simulink model "linear_model"  (R2018b)
settings: Solver=VariableStepAuto  StartTime=0.0  StopTime=5  RelTol=1e-3
values from neighbouring files (symbols this model uses):
  A = [A11 A12 ... (first row only)    [makeBikeModel.m]
  B = [B11 B12 ... (first row only)    [makeBikeModel.m]
  C = eye(2)    [makeBikeModel.m]
  D = 0    [makeBikeModel.m]
  Lf = 2.56    [makeBikeModel.m]    (also in makePlants.m; tunePIDs.m = 0.55)
  Lr = 1.02    [makeBikeModel.m]    (also in makePlants.m; tunePIDs.m = 0.525)
libraries: simulink x1
settings Model: Creator=lachc  LastModifiedBy=lachc

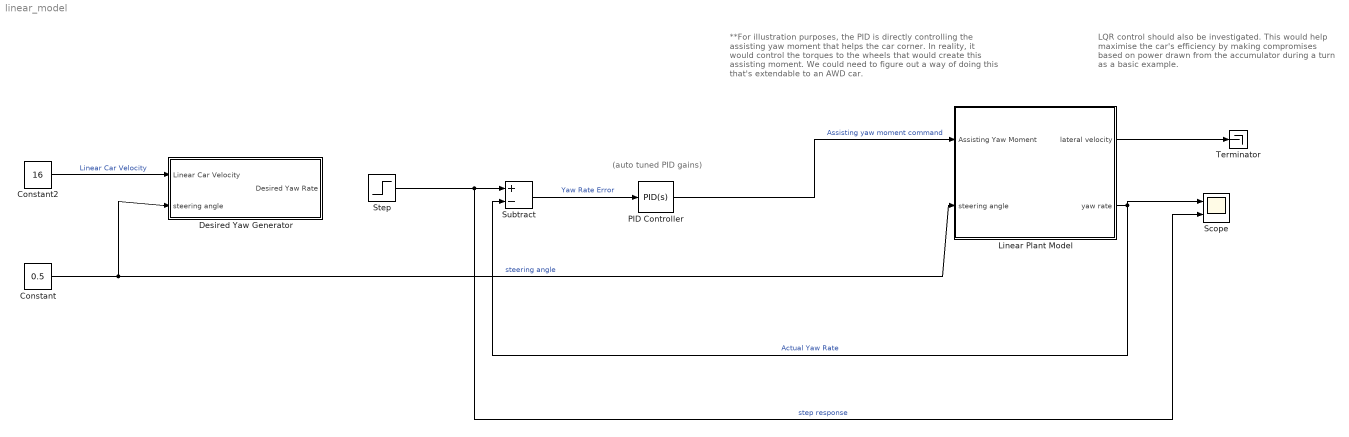
== system linear_model ==
  note: LQR control should also be investigated. This would help maximise the car's efficiency by making compromises based on power drawn from the accumulator during a turn as a basic example.
  note: **For illustration purposes, the PID is directly controlling the assisting yaw moment that helps the car corner. In reality, it would control the torques to the wheels that would create this assisting moment. We could need to figure out a way of doing this that's extendable to an AWD car.
  note: (auto tuned PID gains)
  Constant : Constant  Value=0.5
  Constant2 : Constant  Value=16
  Desired Yaw Generator : Subsystem
  Linear Plant Model : Subsystem
  PID Controller : simulink/Continuous/PID Controller  Controller=PID  Form=Parallel  TimeDomain=Continuous-time  SampleTime=-1  IntegratorMethod=Forward Euler  FilterMethod=Forward Euler  ControllerParametersSource=internal  P=140  I=2312  D=0.85  UseFilter=on  N=47  TunerSelectOption=Transfer Function Based (PID Tuner App)  InitialConditionSource=internal  InitialConditionForIntegrator=0  InitialConditionForFilter=0  DifferentiatorICPrevScaledInput=0  ExternalReset=none  TrackingMode=off  Kt=1  LimitOutput=off  UpperSaturationLimit=inf  LowerSaturationLimit=-inf  LinearizeAsGain=on  AntiWindupMode=none  Kb=1  POutMin=[]  POutMax=[]  IOutMin=[]  IOutMax=[]  DOutMin=[]  DOutMax=[]  NOutMin=[]  NOutMax=[]  SumOutMin=[]  SumOutMax=[]  SaturationOutMin=[]  SaturationOutMax=[]  PParamMin=[]  PParamMax=[]  IParamMin=[]  IParamMax=[]  DParamMin=[]  DParamMax=[]  NParamMin=[]  NParamMax=[]  KbParamMin=[]  KbParamMax=[]  KtParamMin=[]  KtParamMax=[]  KbOutMin=[]  KbOutMax=[]  KtOutMin=[]  KtOutMax=[]  IntegratorOutMin=[]  IntegratorOutMax=[]  FilterOutMin=[]  FilterOutMax=[]  SumI1OutMin=[]  SumI1OutMax=[]  SumI2OutMin=[]  SumI2OutMax=[]  SumI3OutMin=[]  SumI3OutMax=[]  SumI4OutMin=[]  SumI4OutMax=[]  SumDOutMin=[]  SumDOutMax=[]  DifferentiatorOutMin=[]  DifferentiatorOutMax=[]  FilterDiffOutCoefMin=[]  FilterDiffOutCoefMax=[]  ReciprocalOutMin=[]  ReciprocalOutMax=[]  SumDenOutMin=[]  SumDenOutMax=[]  SumNumOutMin=[]  SumNumOutMax=[]  DivideOutMin=[]  DivideOutMax=[]  IntegratorContinuousStateAttributes=''  IntegratorStateMustResolveToSignalObject=off  IntegratorRTWStateStorageClass=Auto  FilterContinuousStateAttributes=''  FilterStateMustResolveToSignalObject=off  FilterRTWStateStorageClass=Auto  ParallelPVariant=InternalParameters  IdealPVariant=Disabled  IVariant=InternalParameters  DVariant=InternalParameters  IntegratorVariant=Continuous  SatVariant=Disabled  AWVariant=Passthrough  PCopyVariant=Disabled  TRVariant=Disabled  FdbkBlocksVariant=Forward  IdealPFdbkVariant=Disabled  SatFdbkVariant=Disabled  DerivativeFilterVariant=ContFilter  NVariant=InternalParameters  NCopyVariant=Disabled  FilterICVariant=InternalICsFilter  IntegratorICVariant=InternalICs  ExternalResetVariant=Disabled  TRSumVariant=Passthrough  SumFdbkVariant=Disabled  SumVariant=Sum_PID
  Scope : Scope  NumInputPorts=2
  Step : Step  After=2  SampleTime=0
  Subtract : Sum  Inputs=+-
  Terminator : Terminator
  wires:
  Linear Plant Model/1(lateral velocity) -> Terminator/1
  Constant2/1 -> Desired Yaw Generator/1(Linear Car Velocity)  "Linear Car Velocity"
  Constant/1 -> Linear Plant Model/2(steering angle), Desired Yaw Generator/2(steering angle)  "steering angle"
  Linear Plant Model/2(yaw rate) -> Subtract/2, Scope/1  "Actual Yaw Rate"
  Subtract/1 -> PID Controller/1  "Yaw Rate Error"
  PID Controller/1 -> Linear Plant Model/1(Assisting Yaw Moment)  "Assisting yaw moment command"
  Step/1 -> Scope/2, Subtract/1  "step response"

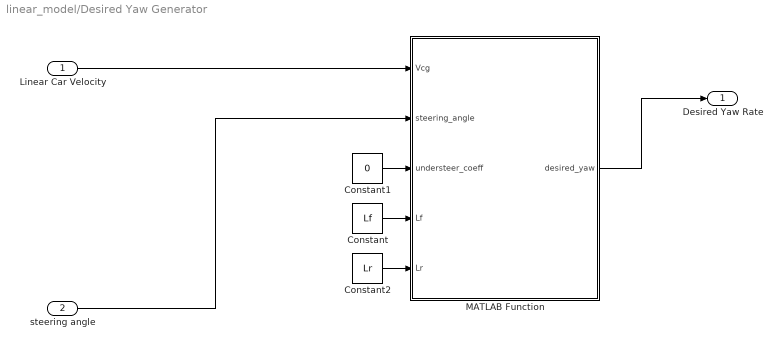
== system linear_model/Desired Yaw Generator ==
  Linear Car Velocity : Inport
  steering angle : Inport  Port=2
  Constant : Constant  Value=Lf
  Constant1 : Constant  Value=0
  Constant2 : Constant  Value=Lr
  MATLAB Function : MATLAB Function  TreatAsAtomicUnit=on
  Desired Yaw Rate : Outport
  wires:
  Constant1/1 -> MATLAB Function/3(understeer_coeff)
  steering angle/1 -> MATLAB Function/2(steering_angle)
  MATLAB Function/1(desired_yaw) -> Desired Yaw Rate/1
  Linear Car Velocity/1 -> MATLAB Function/1(Vcg)
  Constant2/1 -> MATLAB Function/5(Lr)
  Constant/1 -> MATLAB Function/4(Lf)

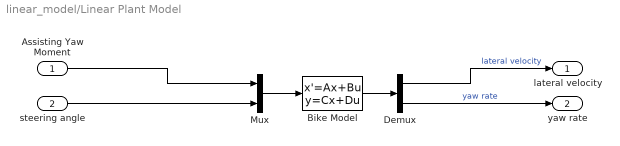
== system linear_model/Linear Plant Model ==
  Assisting Yaw Moment : Inport
  steering angle : Inport  Port=2
  Bike Model : StateSpace  A=A  B=B  C=C  D=D  InitialCondition=0  ContinuousStateAttributes={'V_lat','yaw_rate'}
  Demux : Demux  Outputs=2
  Mux : Mux  Inputs=2
  lateral velocity : Outport
  yaw rate : Outport  Port=2
  wires:
  steering angle/1 -> Mux/2
  Bike Model/1 -> Demux/1
  Demux/2 -> yaw rate/1  "yaw rate"
  Assisting Yaw Moment/1 -> Mux/1
  Mux/1 -> Bike Model/1
  Demux/1 -> lateral velocity/1  "lateral velocity"

== matlab function linear_model/Desired Yaw Generator/MATLAB Function ==
  data: Vcg input; desired_yaw output; steering_angle input; understeer_coeff input; Lf input; Lr input
function desired_yaw = desiredYaw(Vcg , steering_angle, understeer_coeff, Lf, Lr)
desired_yaw = 0;
desired_yaw = Vcg*steering_angle/((Lf*Lr) + understeer_coeff*Vcg^2);
